simulink model "sampleModel172"  (R2021b)
settings: Solver=VariableStepAuto  StartTime=0.0  StopTime=10.0  RelTol=1e-3
undefined symbols (not defined in the file or in its folder): DiscIntNeverNeededParam, magnitude, Newton, Raphson
libraries: simulink x15, slpidlib x2
settings Model: Creator=user  LastModifiedBy=user

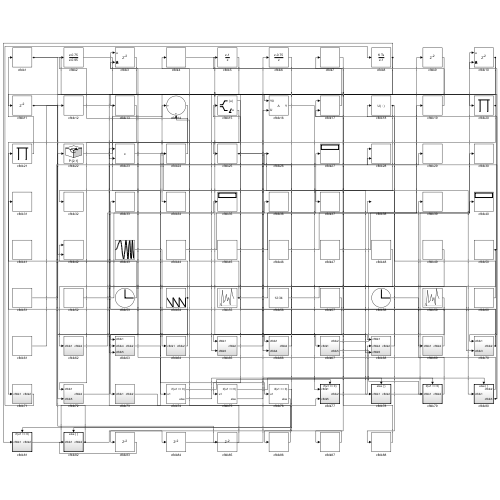
[thumbnail: Simulink's stored preview of the top-level diagram]
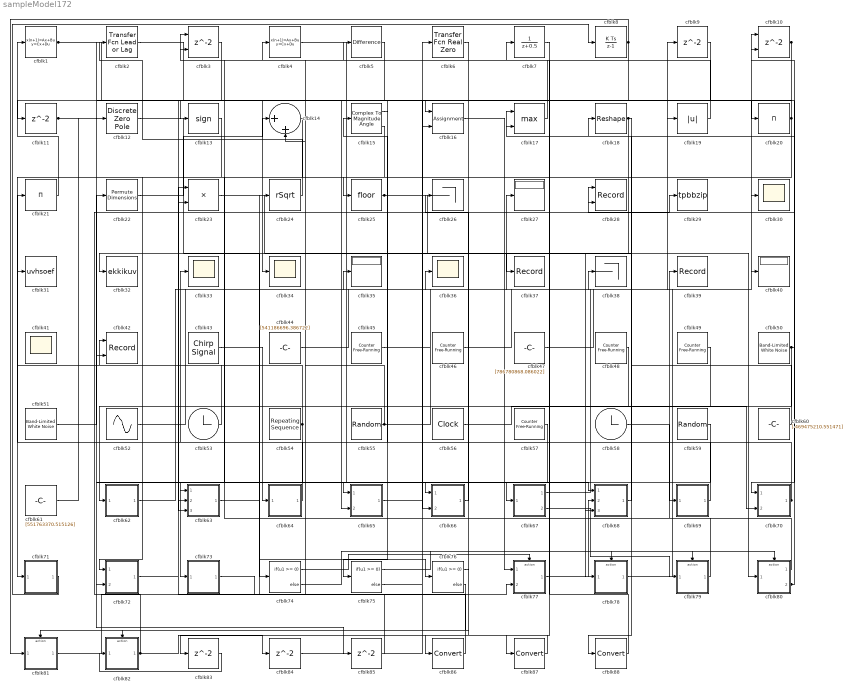
== system sampleModel172 ==
  cfblk1 : DiscreteStateSpace
  cfblk10 : Delay  ShowEnablePort=on  SampleTime=1
      settings: InputPortMap=u0,e6
  cfblk{9,11,83..85} (5 alike) : Delay  SampleTime=1
  cfblk12 : DiscreteZeroPole  Poles=[0 0.5]  Gain=1
  cfblk13 : Signum
  cfblk14 : Sum  Inputs=|++
  cfblk15 : ComplexToMagnitudeAngle
  cfblk16 : Assignment  DiagnosticForDimensions=Warning  IndexOptions=Index vector (dialog)  Indices=1  OutputSizes=1
  cfblk17 : MinMax  Function=max  Inputs=2
  cfblk18 : Reshape
  cfblk19 : Abs
  cfblk2 : simulink/Discrete/Transfer Fcn Lead or Lag  PoleZ=0.95  ZeroZ=0.75  ICPrevOutput=0.0  ICPrevInput=0.0  DoSatur=off
      settings: SourceProductBaseCode=SL
  cfblk20 : Product  Inputs=*
  cfblk21 : Product  Inputs=*
  cfblk22 : PermuteDimensions
  cfblk23 : Product
  cfblk24 : Sqrt  Operator=rSqrt  AlgorithmType=Newton-Raphson  SaturateOnIntegerOverflow=on
  cfblk25 : Rounding
  cfblk26 : Terminator
  cfblk27 : Display
  cfblk28 : Record  FileSettingsInternal="{\"entries\":[{\"content\":{\"excelSettings\":{\"content\":{},\"type\":\"Streamout.ExcelSettings\"}},\"type\":\"Streamout.FileSettingStorage\",\"uuid\":\"4c37d5fb-74dd-4696-a0df-e90e5f7933c2\"}],\"packageUris\":[\"http://schema.mathworks.com/mf0/streamout_blocks/R2020a\"],\"version\":\"1.0\"}"  Layout=[1 1]  SignalsInternal="{\"entries\":[{\"content\":{\"signals\":[{\"content\":{\"blockPath\":[\"sampleModel172/cfblk28\"],\"channel\":[],\"dimensions\":[1],\"domain\":\"sampleModel172/cfblk28\",\"lineColor\":\"#a2142f\",\"plots\":[1],\"port\":1,\"sid\":[\"\"],\"signalID\":6399,\"signalName\":\"cfblk72\"},\"type\":\"RecordBlkView.Signal\",\"uuid\":\"18b58ef6-f147-4f00-97dd-6c5d7728baf2\"},{\"content\":{\"blockPath\":[\"sampleModel172/cfblk28\"],\"channel\":[],\"dimensions\":[1],\"domain\":\"sampleModel172/cfblk28\",\"lineColor\":\"#139fff\",\"plots\":[1],\"port\":2,\"sid\":[\"\"],\"signalID\":6403,\"signalName\":\"cfblk80:2\"},\"type\":\"RecordBlkView.Signal\",\"uuid\":\"a143379a-4b1c-4919-b815-4321dbaf0a81\"}]},\"type\":\"RecordBlkView.InputSignals\",\"uuid\":\"a650f0e4-df4b-47fd-b08d-dcaa5bacfb5c\"}],\"packageUris\":[\"http://schema.mathworks.com/mf0/streamout_blocks/R2020a\"],\"version\":\"1.0\"}"  VisualizationBindings="{\"xyplotplugin\":{\"info\":[{\"series\":[{\"bindingParametersList\":[{\"parameter\":\"X-Axis\",\"signalID\":6399,\"signalName\":\"cfblk72\"},{\"parameter\":\"Y-Axis\",\"signalID\":6403,\"signalName\":\"cfblk80:2\"}],\"seriesID\":36726}],\"subplotID\":1}]}}"  CompatibilityTag=XY
  cfblk29 : ToWorkspace  VariableName=tpbbzip  SaveFormat=Timeseries  SampleTime=-1
  cfblk3 : Delay  ShowEnablePort=on  SampleTime=1
      settings: InputPortMap=u0,e6
  cfblk{30,33..34,36,41} (5 alike) : Scope
      cfblk41 settings: Floating=on
  cfblk31 : ToWorkspace  VariableName=uvhsoef  SaveFormat=Timeseries  SampleTime=-1
  cfblk32 : ToWorkspace  VariableName=ekkikuv  SaveFormat=Timeseries  SampleTime=-1
  cfblk35 : Display
  cfblk37 : Record  FileSettingsInternal="{\"entries\":[{\"content\":{\"excelSettings\":{\"content\":{},\"type\":\"Streamout.ExcelSettings\"}},\"type\":\"Streamout.FileSettingStorage\",\"uuid\":\"666d1965-106f-49f3-aa2f-b556bec9c068\"}],\"packageUris\":[\"http://schema.mathworks.com/mf0/streamout_blocks/R2020a\"],\"version\":\"1.0\"}"  SignalsInternal="{\"entries\":[{\"content\":{\"signals\":[{\"content\":{\"blockPath\":[\"sampleModel172/cfblk37\"],\"channel\":[],\"dimensions\":[1],\"domain\":\"sampleModel172/cfblk37\",\"lineColor\":\"#64d413\",\"plots\":[1],\"port\":1,\"sid\":[\"\"],\"signalID\":6409,\"signalName\":\"cfblk18\"},\"type\":\"RecordBlkView.Signal\",\"uuid\":\"579457c8-c496-41a4-82c2-eba13d432ecc\"}]},\"type\":\"RecordBlkView.InputSignals\",\"uuid\":\"6e0c83c2-8fe5-488b-bd7b-1d63ca069db9\"}],\"packageUris\":[\"http://schema.mathworks.com/mf0/streamout_blocks/R2020a\"],\"version\":\"1.0\"}"  VisualizationBindings="{\"sparklinesplugin\":{\"info\":[{\"bindingParametersList\":[],\"subplotID\":1}]}}"
  cfblk38 : Terminator
  cfblk39 : Record  FileSettingsInternal="{\"entries\":[{\"content\":{\"excelSettings\":{\"content\":{},\"type\":\"Streamout.ExcelSettings\"}},\"type\":\"Streamout.FileSettingStorage\",\"uuid\":\"d348c3f3-15d7-45a7-9944-3cee22ff94f9\"}],\"packageUris\":[\"http://schema.mathworks.com/mf0/streamout_blocks/R2020a\"],\"version\":\"1.0\"}"  SignalsInternal="{\"entries\":[{\"content\":{\"signals\":[{\"content\":{\"blockPath\":[\"sampleModel172/cfblk39\"],\"channel\":[],\"dimensions\":[1],\"domain\":\"sampleModel172/cfblk39\",\"lineColor\":\"#ff13a6\",\"plots\":[1],\"port\":1,\"sid\":[\"\"],\"signalID\":6413,\"signalName\":\"cfblk79\"},\"type\":\"RecordBlkView.Signal\",\"uuid\":\"ee09b67d-d6f4-4d50-be6d-3dddccd276d5\"}]},\"type\":\"RecordBlkView.InputSignals\",\"uuid\":\"6358c080-dbab-4218-a449-23edf1143d2e\"}],\"packageUris\":[\"http://schema.mathworks.com/mf0/streamout_blocks/R2020a\"],\"version\":\"1.0\"}"  VisualizationBindings="{\"sparklinesplugin\":{\"info\":[{\"bindingParametersList\":[],\"subplotID\":1}]}}"
  cfblk4 : DiscreteStateSpace
  cfblk40 : Display
  cfblk42 : Record  FileSettingsInternal="{\"entries\":[{\"content\":{\"excelSettings\":{\"content\":{},\"type\":\"Streamout.ExcelSettings\"}},\"type\":\"Streamout.FileSettingStorage\",\"uuid\":\"79f54138-a6c4-42fd-9433-9cd93f3ff392\"}],\"packageUris\":[\"http://schema.mathworks.com/mf0/streamout_blocks/R2020a\"],\"version\":\"1.0\"}"  Layout=[1 1]  SignalsInternal="{\"entries\":[{\"content\":{\"signals\":[{\"content\":{\"blockPath\":[\"sampleModel172/cfblk42\"],\"channel\":[],\"dimensions\":[1],\"domain\":\"sampleModel172/cfblk42\",\"lineColor\":\"#a2142f\",\"plots\":[1],\"port\":1,\"sid\":[\"\"],\"signalID\":6417,\"signalName\":\"cfblk54\"},\"type\":\"RecordBlkView.Signal\",\"uuid\":\"99384b5f-59da-4b0b-b0ff-6a1d5a9a7f91\"},{\"content\":{\"blockPath\":[\"sampleModel172/cfblk42\"],\"channel\":[],\"dimensions\":[1],\"domain\":\"sampleModel172/cfblk42\",\"lineColor\":\"#139fff\",\"plots\":[1],\"port\":2,\"sid\":[\"\"],\"signalID\":6421,\"signalName\":\"cfblk8\"},\"type\":\"RecordBlkView.Signal\",\"uuid\":\"effeabc5-6d8e-48d5-a229-b5f369d7cadd\"}]},\"type\":\"RecordBlkView.InputSignals\",\"uuid\":\"76116694-bd45-480f-96f3-05638feb9283\"}],\"packageUris\":[\"http://schema.mathworks.com/mf0/streamout_blocks/R2020a\"],\"version\":\"1.0\"}"  VisualizationBindings="{\"xyplotplugin\":{\"info\":[{\"series\":[{\"bindingParametersList\":[{\"parameter\":\"X-Axis\",\"signalID\":6417,\"signalName\":\"cfblk54\"},{\"parameter\":\"Y-Axis\",\"signalID\":6421,\"signalName\":\"cfblk8\"}],\"seriesID\":3961}],\"subplotID\":1}]}}"  CompatibilityTag=XY
  cfblk43 : simulink/Sources/Chirp Signal  f1=[-247826530.279235]  T=[-723031258.847679]  f2=[-950914322.250335]
  cfblk44 : Constant  Value=[541186696.386722]  SampleTime=1
  cfblk45 : simulink/Sources/Counter Free-Running  NumBits=[26.000000]  tsamp=-1
  cfblk46 : simulink/Sources/Counter Free-Running  NumBits=[21.000000]  tsamp=-1
  cfblk47 : Constant  Value=[786780868.086022]  SampleTime=1
  cfblk48 : simulink/Sources/Counter Free-Running  NumBits=[26.000000]  tsamp=-1
  cfblk49 : simulink/Sources/Counter Free-Running  NumBits=[24.000000]  tsamp=-1
  cfblk5 : simulink/Discrete/Difference  ICPrevInput=0.0  OutMin=[]  OutMax=[]  OutDataTypeStr=Inherit: Inherit via back propagation  OutDataType=fixdt(1, 16)  OutScaling=2^-10  DoSatur=off
  cfblk50 : simulink/Sources/Band-Limited White Noise  Cov=[3939442188.856112]  Ts=0.1  seed=[8004305238.000000]
  cfblk51 : simulink/Sources/Band-Limited White Noise  Cov=[506599525.113534]  Ts=0.1  seed=[1350061790.000000]
  cfblk52 : Sin  Amplitude=[-381260761.661942]  Bias=[134835104.739763]  SampleTime=0
  cfblk53 : Clock
  cfblk54 : simulink/Sources/Repeating Sequence  rep_seq_t=[0 2]  rep_seq_y=[-269044501.698545, -539833890.638024]
  cfblk55 : UniformRandomNumber  Minimum=[-2930461244.017724]  Maximum=[2395720489.749123]  Seed=[78690133.000000]  SampleTime=0.1
  cfblk56 : DigitalClock
  cfblk57 : simulink/Sources/Counter Free-Running  NumBits=[38.000000]  tsamp=-1
  cfblk58 : Clock
  cfblk59 : UniformRandomNumber  Minimum=[-3055983286.462450]  Maximum=[6128316988.201324]  Seed=[15339092.000000]  SampleTime=0.1
  cfblk6 : simulink/Discrete/Transfer Fcn Real Zero  ZeroZ=0.75  ICPrevInput=0.0  DoSatur=off
      settings: SourceProductBaseCode=SL
  cfblk60 : Constant  Value=[-469475210.551471]  SampleTime=1
  cfblk61 : Constant  Value=[551763370.515126]  SampleTime=1
  cfblk62 : Subsystem
  cfblk63 : Subsystem
  cfblk64 : Subsystem
  cfblk65 : Subsystem
  cfblk66 : Subsystem
  cfblk67 : Subsystem
  cfblk68 : Subsystem
  cfblk69 : Subsystem
  cfblk7 : DiscreteTransferFcn  SampleTime=1
  cfblk70 : Subsystem
  cfblk71 : Subsystem
  cfblk72 : Subsystem
  cfblk73 : Subsystem
  cfblk74 : If  IfExpression=u1 >= 0  SampleTime=1
  cfblk75 : If  IfExpression=u1 >= 0  SampleTime=1
  cfblk76 : If  IfExpression=u1 >= 0  SampleTime=1
  cfblk77 : Subsystem  TreatAsAtomicUnit=on
  cfblk78 : Subsystem  TreatAsAtomicUnit=on
  cfblk79 : Subsystem  TreatAsAtomicUnit=on
  cfblk8 : DiscreteIntegrator  ICPrevOutput=DiscIntNeverNeededParam  ICPrevScaledInput=DiscIntNeverNeededParam
  cfblk80 : Subsystem  TreatAsAtomicUnit=on
  cfblk81 : Subsystem  TreatAsAtomicUnit=on
  cfblk82 : Subsystem  TreatAsAtomicUnit=on
  cfblk86 : DataTypeConversion
  cfblk87 : DataTypeConversion
  cfblk88 : DataTypeConversion
  wires:
  cfblk59/1 -> cfblk73/1(cfblk1)
  cfblk62/1(cfblk2) -> cfblk38/1
  cfblk44/1 -> cfblk36/1
  cfblk60/1 -> cfblk32/1
  cfblk61/1 -> cfblk12/1
  cfblk1/1 -> cfblk70/1(cfblk1), cfblk20/1
  cfblk82/1(cfblk2) -> cfblk29/1, cfblk84/1
  cfblk55/1 -> cfblk27/1, cfblk14/2
  cfblk56/1 -> cfblk70/2(cfblk3)
  cfblk51/1 -> cfblk22/1
  cfblk21/1 -> cfblk1/1
  cfblk14/1 -> cfblk71/1(cfblk1)
  cfblk16/1 -> cfblk77/1(cfblk1)
  cfblk24/1 -> cfblk2/1
  cfblk10/1 -> cfblk34/1, cfblk25/1
  cfblk64/1(cfblk2) -> cfblk33/1
  cfblk57/1 -> cfblk65/1(cfblk1)
  cfblk79/1(cfblk2) -> cfblk39/1
  cfblk2/1 -> cfblk16/1
  cfblk43/1 -> cfblk64/1(cfblk1)
  cfblk47/1 -> cfblk9/1
  cfblk12/1 -> cfblk74/1
  cfblk19/1 -> cfblk3/1
  cfblk13/1 -> cfblk72/1(cfblk1)
  cfblk15/1 -> cfblk75/1
  cfblk4/1 -> cfblk67/1(cfblk1)
  cfblk20/1 -> cfblk13/1, cfblk23/2
  cfblk67/1(cfblk2) -> cfblk10/1
  cfblk78/1(cfblk2) -> cfblk30/1
  cfblk72/1(cfblk2) -> cfblk28/1
  cfblk15/2 -> cfblk63/1(cfblk1)
  cfblk50/1 -> cfblk63/2(cfblk4), cfblk10/2
  cfblk9/1 -> cfblk65/2(cfblk5)
  cfblk52/1 -> cfblk35/1
  cfblk73/1(cfblk2) -> cfblk77/2(cfblk5)
  cfblk71/1(cfblk2) -> cfblk8/1
  cfblk11/1 -> cfblk68/1(cfblk1), cfblk85/1
  cfblk80/1(cfblk2) -> cfblk3/2
  cfblk77/1(cfblk2) -> cfblk68/2(cfblk4)
  cfblk63/1(cfblk2) -> cfblk76/1
  cfblk23/1 -> cfblk80/1(cfblk1)
  cfblk68/1(cfblk2) -> cfblk18/1
  cfblk67/2(cfblk5) -> cfblk79/1(cfblk1)
  cfblk46/1 -> cfblk40/1
  cfblk5/1 -> cfblk63/3(cfblk5)
  cfblk18/1 -> cfblk37/1, cfblk88/1
  cfblk54/1 -> cfblk72/2(cfblk5), cfblk42/1
  cfblk25/1 -> cfblk78/1(cfblk1), cfblk68/3(cfblk5)
  cfblk45/1 -> cfblk19/1
  cfblk81/1(cfblk2) -> cfblk24/1
  cfblk8/1 -> cfblk81/1(cfblk1), cfblk66/2(cfblk4), cfblk42/2
  cfblk48/1 -> cfblk62/1(cfblk1)
  cfblk58/1 -> cfblk69/1(cfblk1)
  cfblk69/1(cfblk2) -> cfblk15/1
  cfblk3/1 -> cfblk11/1
  cfblk6/1 -> cfblk66/1(cfblk1)
  cfblk53/1 -> cfblk21/1
  cfblk22/1 -> cfblk14/1
  cfblk66/1(cfblk2) -> cfblk26/1
  cfblk70/1(cfblk2) -> cfblk17/1, cfblk31/1
  cfblk17/1 -> cfblk5/1
  cfblk65/1(cfblk2) -> cfblk6/1
  cfblk80/2(cfblk3) -> cfblk28/2, cfblk17/2
  cfblk74/1 -> cfblk77/Action
  cfblk74/2 -> cfblk78/Action
  cfblk75/1 -> cfblk79/Action
  cfblk75/2 -> cfblk80/Action
  cfblk76/1 -> cfblk81/Action
  cfblk76/2 -> cfblk82/Action
  cfblk83/1 -> cfblk82/1(cfblk1)
  cfblk84/1 -> cfblk16/2
  cfblk85/1 -> cfblk23/1
  cfblk49/1 -> cfblk86/1
  cfblk86/1 -> cfblk4/1
  cfblk7/1 -> cfblk87/1
  cfblk87/1 -> cfblk83/1
  cfblk88/1 -> cfblk7/1

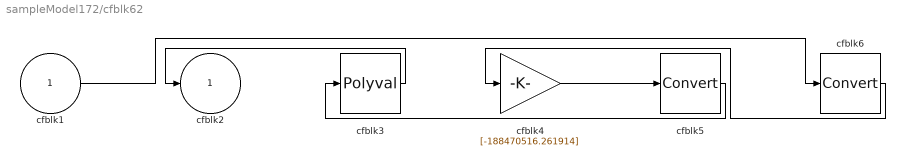
== system sampleModel172/cfblk62 ==
  cfblk1 : Inport
  cfblk3 : Polyval  Coefs=[ +2.081618890e-019, -1.441693666e-014, +4.719686976e-010, -8.536869453e-006, +1.621573104e-001, -8.087801117e+001 ]
  cfblk4 : Gain  Gain=[-188470516.261914]
  cfblk5 : DataTypeConversion
  cfblk6 : DataTypeConversion
  cfblk2 : Outport
  wires:
  cfblk3/1 -> cfblk2/1
  cfblk4/1 -> cfblk5/1
  cfblk5/1 -> cfblk3/1
  cfblk1/1 -> cfblk6/1
  cfblk6/1 -> cfblk4/1

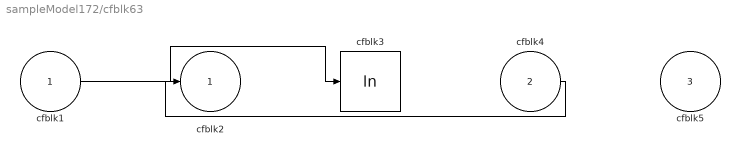
== system sampleModel172/cfblk63 ==
  cfblk1 : Inport
  cfblk4 : Inport  Port=2
  cfblk5 : Inport  Port=3
  cfblk3 : Math  Operator=log  SaturateOnIntegerOverflow=on
  cfblk2 : Outport
  wires:
  cfblk1/1 -> cfblk3/1
  cfblk4/1 -> cfblk2/1

== system sampleModel172/cfblk64 ==
  cfblk1 : Inport
  cfblk3 : DotProduct  InputSameDT=on  OutDataTypeStr=Inherit: Inherit via internal rule
  cfblk2 : Outport
  wires:
  cfblk1/1 -> cfblk3/1, cfblk3/2
  cfblk3/1 -> cfblk2/1

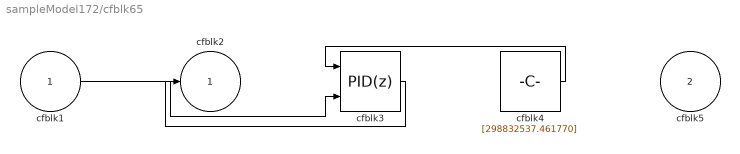
== system sampleModel172/cfblk65 ==
  cfblk1 : Inport
  cfblk5 : Inport  Port=2
  cfblk3 : slpidlib/PID Controller (2DOF)  Controller=PID  Form=Parallel  TimeDomain=Discrete-time  UseExternalTs=off  SampleTime=1  IntegratorMethod=Forward Euler  FilterMethod=Forward Euler  ControllerParametersSource=internal  P=1  I=1  D=0  UseFilter=on  N=100  b=1  c=1  TunerSelectOption=Transfer Function Based (PID Tuner App)  InitialConditionSource=internal  InitialConditionForIntegrator=0  InitialConditionForFilter=0  DifferentiatorICPrevScaledInput=0  ExternalReset=none  TrackingMode=off  Kt=1  LimitOutput=off  SatLimitsSource=internal  UpperSaturationLimit=inf  LowerSaturationLimit=-inf  LinearizeAsGain=off  AntiWindupMode=none  Kb=1  POutMin=[]  POutMax=[]  IOutMin=[]  IOutMax=[]  DOutMin=[]  DOutMax=[]  NOutMin=[]  NOutMax=[]  bOutMin=[]  bOutMax=[]  cOutMin=[]  cOutMax=[]  SumOutMin=[]  SumOutMax=[]  SaturationOutMin=[]  SaturationOutMax=[]  PParamMin=[]  PParamMax=[]  IParamMin=[]  IParamMax=[]  DParamMin=[]  DParamMax=[]  NParamMin=[]  NParamMax=[]  bParamMin=[]  bParamMax=[]  cParamMin=[]  cParamMax=[]  KbParamMin=[]  KbParamMax=[]  KtParamMin=[]  KtParamMax=[]  KbOutMin=[]  KbOutMax=[]  KtOutMin=[]  KtOutMax=[]  IntegratorOutMin=[]  IntegratorOutMax=[]  FilterOutMin=[]  FilterOutMax=[]  SumI1OutMin=[]  SumI1OutMax=[]  SumI2OutMin=[]  SumI2OutMax=[]  SumI3OutMin=[]  SumI3OutMax=[]  SumI4OutMin=[]  SumI4OutMax=[]  SumDOutMin=[]  SumDOutMax=[]  Sum1OutMin=[]  Sum1OutMax=[]  Sum2OutMin=[]  Sum2OutMax=[]  Sum3OutMin=[]  Sum3OutMax=[]  DifferentiatorOutMin=[]  DifferentiatorOutMax=[]  FilterDiffOutCoefMin=[]  FilterDiffOutCoefMax=[]  ReciprocalOutMin=[]  ReciprocalOutMax=[]  SumDenOutMin=[]  SumDenOutMax=[]  SumNumOutMin=[]  SumNumOutMax=[]  DivideOutMin=[]  DivideOutMax=[]  UdiffTsProdOutMin=[]  UdiffTsProdOutMax=[]  NTsProdOutMin=[]  NTsProdOutMax=[]  UintegralTsProdOutMin=[]  UintegralTsProdOutMax=[]  UngainTsProdOutMin=[]  UngainTsProdOutMax=[]  IntegratorContinuousStateAttributes=''  IntegratorStateMustResolveToSignalObject=off  IntegratorRTWStateStorageClass=Auto  FilterContinuousStateAttributes=''  FilterStateMustResolveToSignalObject=off  FilterRTWStateStorageClass=Auto  ParallelPVariant=InternalParameters  IdealPVariant=Disabled  IVariant=InternalParameters  DVariant=InternalParameters  bVariant=InternalParameters  cVariant=InternalParameters  IntegratorVariant=Discrete  SatVariant=Disabled  AWVariant=Passthrough  PCopyVariant=Disabled  TRVariant=Disabled  FdbkBlocksVariant=Forward  IdealPFdbkVariant=Disabled  SatFdbkVariant=Disabled  DerivativeFilterVariant=ForwardEulerFilter  NVariant=InternalParameters  NCopyVariant=Disabled  FilterICVariant=InternalICsFilter  IntegratorICVariant=InternalICs  ExternalResetVariant=Disabled  TRSumVariant=Passthrough  SumFdbkVariant=Disabled  SumVariant=Sum_PID  TsampFilterVariant=InternalTs  TsampNgainVariant=Passthrough  TsampIntegralVariant=Passthrough  ExternalSaturationOutDataTypeStr=Inherit: Same as second input
      settings: SourceProductBaseCode=SL
  cfblk4 : Constant  Value=[298832537.461770]  SampleTime=1
  cfblk2 : Outport
  wires:
  cfblk4/1 -> cfblk3/1
  cfblk1/1 -> cfblk3/2
  cfblk3/1 -> cfblk2/1

== system sampleModel172/cfblk66 ==
  cfblk1 : Inport
  cfblk4 : Inport  Port=2
  cfblk3 : DiscreteFir  SampleTime=1
  cfblk2 : Outport
  wires:
  cfblk4/1 -> cfblk2/1
  cfblk1/1 -> cfblk3/1

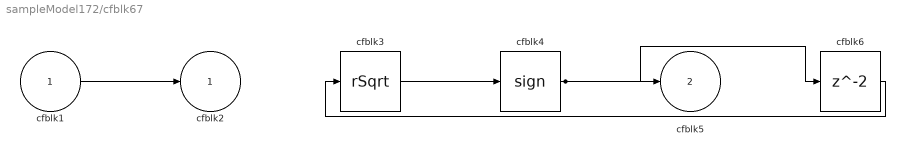
== system sampleModel172/cfblk67 ==
  cfblk1 : Inport
  cfblk3 : Sqrt  Operator=rSqrt  AlgorithmType=Newton-Raphson  SaturateOnIntegerOverflow=on
  cfblk4 : Signum
  cfblk6 : Delay  SampleTime=1
  cfblk2 : Outport
  cfblk5 : Outport  Port=2
  wires:
  cfblk4/1 -> cfblk5/1, cfblk6/1
  cfblk3/1 -> cfblk4/1
  cfblk1/1 -> cfblk2/1
  cfblk6/1 -> cfblk3/1

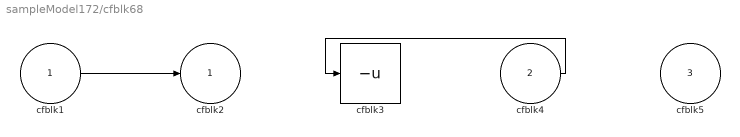
== system sampleModel172/cfblk68 ==
  cfblk1 : Inport
  cfblk4 : Inport  Port=2
  cfblk5 : Inport  Port=3
  cfblk3 : UnaryMinus
  cfblk2 : Outport
  wires:
  cfblk1/1 -> cfblk2/1
  cfblk4/1 -> cfblk3/1

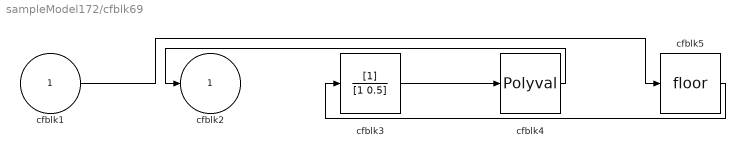
== system sampleModel172/cfblk69 ==
  cfblk1 : Inport
  cfblk3 : DiscreteFilter  SampleTime=1
  cfblk4 : Polyval  Coefs=[ +2.081618890e-019, -1.441693666e-014, +4.719686976e-010, -8.536869453e-006, +1.621573104e-001, -8.087801117e+001 ]
  cfblk5 : Rounding
  cfblk2 : Outport
  wires:
  cfblk4/1 -> cfblk2/1
  cfblk5/1 -> cfblk3/1
  cfblk3/1 -> cfblk4/1
  cfblk1/1 -> cfblk5/1

== system sampleModel172/cfblk70 ==
  cfblk1 : Inport
  cfblk3 : Inport  Port=2
  cfblk2 : Outport
  wires:
  cfblk3/1 -> cfblk2/1

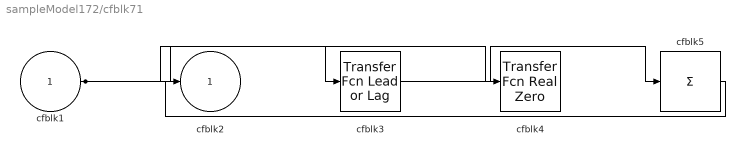
== system sampleModel172/cfblk71 ==
  cfblk1 : Inport
  cfblk3 : simulink/Discrete/Transfer Fcn Lead or Lag  PoleZ=0.95  ZeroZ=0.75  ICPrevOutput=0.0  ICPrevInput=0.0  DoSatur=off
      settings: SourceProductBaseCode=SL
  cfblk4 : simulink/Discrete/Transfer Fcn Real Zero  ZeroZ=0.75  ICPrevInput=0.0  DoSatur=off
      settings: SourceProductBaseCode=SL
  cfblk5 : Sum  Inputs=+
  cfblk2 : Outport
  wires:
  cfblk1/1 -> cfblk3/1, cfblk4/1
  cfblk3/1 -> cfblk5/1
  cfblk5/1 -> cfblk2/1

== system sampleModel172/cfblk72 ==
  cfblk1 : Inport
  cfblk5 : Inport  Port=2
  cfblk3 : slpidlib/PID Controller  Controller=PID  Form=Parallel  TimeDomain=Discrete-time  UseExternalTs=off  SampleTime=1  IntegratorMethod=Forward Euler  FilterMethod=Forward Euler  ControllerParametersSource=internal  P=1  I=1  D=0  UseFilter=on  N=100  TunerSelectOption=Transfer Function Based (PID Tuner App)  InitialConditionSource=internal  InitialConditionForIntegrator=0  InitialConditionForFilter=0  DifferentiatorICPrevScaledInput=0  ExternalReset=none  TrackingMode=off  Kt=1  LimitOutput=off  SatLimitsSource=internal  UpperSaturationLimit=inf  LowerSaturationLimit=-inf  LinearizeAsGain=off  AntiWindupMode=none  Kb=1  POutMin=[]  POutMax=[]  IOutMin=[]  IOutMax=[]  DOutMin=[]  DOutMax=[]  NOutMin=[]  NOutMax=[]  SumOutMin=[]  SumOutMax=[]  SaturationOutMin=[]  SaturationOutMax=[]  PParamMin=[]  PParamMax=[]  IParamMin=[]  IParamMax=[]  DParamMin=[]  DParamMax=[]  NParamMin=[]  NParamMax=[]  KbParamMin=[]  KbParamMax=[]  KtParamMin=[]  KtParamMax=[]  KbOutMin=[]  KbOutMax=[]  KtOutMin=[]  KtOutMax=[]  IntegratorOutMin=[]  IntegratorOutMax=[]  FilterOutMin=[]  FilterOutMax=[]  SumI1OutMin=[]  SumI1OutMax=[]  SumI2OutMin=[]  SumI2OutMax=[]  SumI3OutMin=[]  SumI3OutMax=[]  SumI4OutMin=[]  SumI4OutMax=[]  SumDOutMin=[]  SumDOutMax=[]  DifferentiatorOutMin=[]  DifferentiatorOutMax=[]  FilterDiffOutCoefMin=[]  FilterDiffOutCoefMax=[]  ReciprocalOutMin=[]  ReciprocalOutMax=[]  SumDenOutMin=[]  SumDenOutMax=[]  SumNumOutMin=[]  SumNumOutMax=[]  DivideOutMin=[]  DivideOutMax=[]  UdiffTsProdOutMin=[]  UdiffTsProdOutMax=[]  NTsProdOutMin=[]  NTsProdOutMax=[]  UintegralTsProdOutMin=[]  UintegralTsProdOutMax=[]  UngainTsProdOutMin=[]  UngainTsProdOutMax=[]  IntegratorContinuousStateAttributes=''  IntegratorStateMustResolveToSignalObject=off  IntegratorRTWStateStorageClass=Auto  FilterContinuousStateAttributes=''  FilterStateMustResolveToSignalObject=off  FilterRTWStateStorageClass=Auto  ParallelPVariant=InternalParameters  IdealPVariant=Disabled  IVariant=InternalParameters  DVariant=InternalParameters  IntegratorVariant=Discrete  SatVariant=Disabled  AWVariant=Passthrough  PCopyVariant=Disabled  TRVariant=Disabled  FdbkBlocksVariant=Forward  IdealPFdbkVariant=Disabled  SatFdbkVariant=Disabled  DerivativeFilterVariant=ForwardEulerFilter  NVariant=InternalParameters  NCopyVariant=Disabled  FilterICVariant=InternalICsFilter  IntegratorICVariant=InternalICs  ExternalResetVariant=Disabled  TRSumVariant=Passthrough  SumFdbkVariant=Disabled  SumVariant=Sum_PID  TsampFilterVariant=InternalTs  TsampNgainVariant=Passthrough  TsampIntegralVariant=Passthrough  ExternalSaturationOutDataTypeStr=Inherit: Same as second input
  cfblk4 : Sum
  cfblk2 : Outport
  wires:
  cfblk5/1 -> cfblk3/1, cfblk4/2
  cfblk1/1 -> cfblk4/1
  cfblk3/1 -> cfblk2/1

== system sampleModel172/cfblk73 ==
  cfblk1 : Inport
  cfblk3 : DiscreteIntegrator  ICPrevOutput=DiscIntNeverNeededParam  ICPrevScaledInput=DiscIntNeverNeededParam
  cfblk2 : Outport
  wires:
  cfblk1/1 -> cfblk3/1
  cfblk3/1 -> cfblk2/1

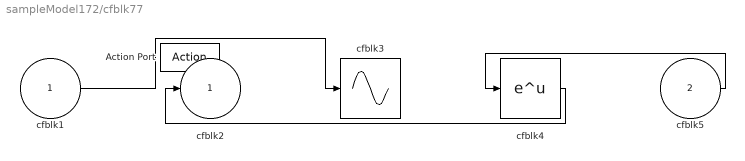
== system sampleModel172/cfblk77 ==
  cfblk1 : Inport
  cfblk5 : Inport  Port=2
  Action Port : ActionPort  ActionPortLabel=if(u1 >= 0)
  cfblk3 : Sin  TimeSource=Use external signal  SampleTime=0
  cfblk4 : Math  SaturateOnIntegerOverflow=on
  cfblk2 : Outport
  wires:
  cfblk4/1 -> cfblk2/1
  cfblk5/1 -> cfblk4/1
  cfblk1/1 -> cfblk3/1

== system sampleModel172/cfblk78 ==
  cfblk1 : Inport
  Action Port : ActionPort  ActionPortLabel=else
  cfblk3 : Sin  TimeSource=Use external signal  SampleTime=0
  cfblk2 : Outport
  wires:
  cfblk1/1 -> cfblk2/1, cfblk3/1

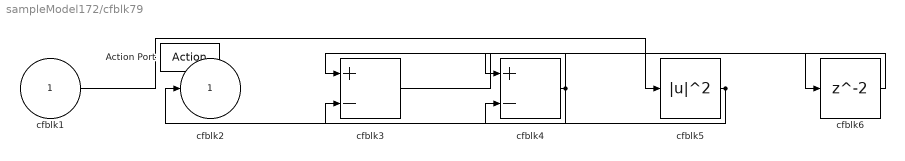
== system sampleModel172/cfblk79 ==
  cfblk1 : Inport
  Action Port : ActionPort  ActionPortLabel=if(u1 >= 0)
  cfblk3 : Sum  Inputs=+-
  cfblk4 : Sum  Inputs=+-
  cfblk5 : Math  Operator=magnitude^2  SaturateOnIntegerOverflow=on
  cfblk6 : Delay
  cfblk2 : Outport
  wires:
  cfblk5/1 -> cfblk4/2, cfblk2/1
  cfblk4/1 -> cfblk3/1, cfblk3/2
  cfblk1/1 -> cfblk5/1
  cfblk3/1 -> cfblk6/1
  cfblk6/1 -> cfblk4/1

== system sampleModel172/cfblk80 ==
  cfblk1 : Inport
  Action Port : ActionPort  ActionPortLabel=else
  cfblk2 : Outport
  cfblk3 : Outport  Port=2
  wires:
  cfblk1/1 -> cfblk2/1, cfblk3/1

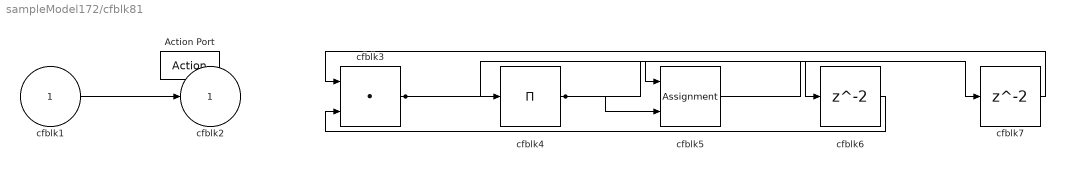
== system sampleModel172/cfblk81 ==
  cfblk1 : Inport
  Action Port : ActionPort  ActionPortLabel=if(u1 >= 0)
  cfblk3 : DotProduct  InputSameDT=on  OutDataTypeStr=Inherit: Inherit via internal rule
  cfblk4 : Product  Inputs=*
  cfblk5 : Assignment  DiagnosticForDimensions=Warning  IndexOptions=Index vector (dialog)  Indices=1  OutputSizes=1
  cfblk6 : Delay
  cfblk7 : Delay
  cfblk2 : Outport
  wires:
  cfblk4/1 -> cfblk5/2, cfblk6/1
  cfblk1/1 -> cfblk2/1
  cfblk3/1 -> cfblk4/1, cfblk5/1
  cfblk6/1 -> cfblk3/2
  cfblk5/1 -> cfblk7/1
  cfblk7/1 -> cfblk3/1

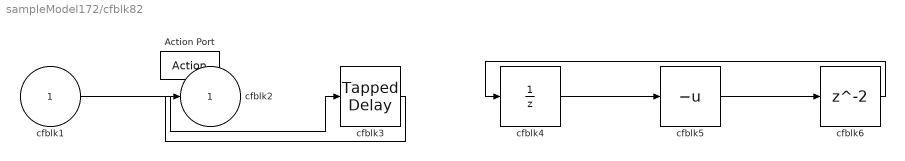
== system sampleModel172/cfblk82 ==
  cfblk1 : Inport
  Action Port : ActionPort  ActionPortLabel=else
  cfblk3 : simulink/Discrete/Tapped Delay  vinit=0.0  samptime=-1  NumDelays=1  DelayOrder=Oldest  includeCurrent=off
  cfblk4 : UnitDelay  SampleTime=-1  HasFrameUpgradeWarning=on
  cfblk5 : UnaryMinus
  cfblk6 : Delay
  cfblk2 : Outport
  wires:
  cfblk1/1 -> cfblk3/1
  cfblk3/1 -> cfblk2/1
  cfblk4/1 -> cfblk5/1
  cfblk5/1 -> cfblk6/1
  cfblk6/1 -> cfblk4/1
